simulink model "Calculate_average"  (R2021a)
settings: Solver=FixedStepDiscrete  StartTime=0.0  StopTime=10.0  RelTol=1e-3
settings Model: Creator=OmarMedhat  LastModifiedBy=OmarMedhat
settings OptimizationCC: DefaultParameterBehavior=Inlined  EnhancedBackFolding=on  PassReuseOutputArgsAs=Individual arguments  ZeroExternalMemoryAtStartup=off  ZeroInternalMemoryAtStartup=off  OptimizeBlockOrder=speed  DifferentSizesBufferReuse=on  OptimizationCustomize=off  EfficientTunableParamExpr=on
settings DebuggingCC: ParameterTunabilityLossMsg=error
settings SFSimCC: MATLABDynamicMemAlloc=off
settings RTWCC: SystemTargetFile=ert.tlc  GenCodeOnly=on  TemplateMakefile=ert_default_tmf  GenerateReport=on  IncludeHyperlinkInReport=on  LaunchReport=on  GenerateTraceInfo=on
settings CodeAppCC: ForceParamTrailComments=on  IgnoreCustomStorageClasses=off  OperatorAnnotations=on  SimulinkDataObjDesc=on  SFDataObjDesc=on  InsertBlockDesc=on
settings ERTTargetCC: TargetLangStandard=C99 (ISO)  GenerateSampleERTMain=on  InlinedParameterPlacement=NonHierarchical  ERTCustomFileTemplate=example_file_process.tlc

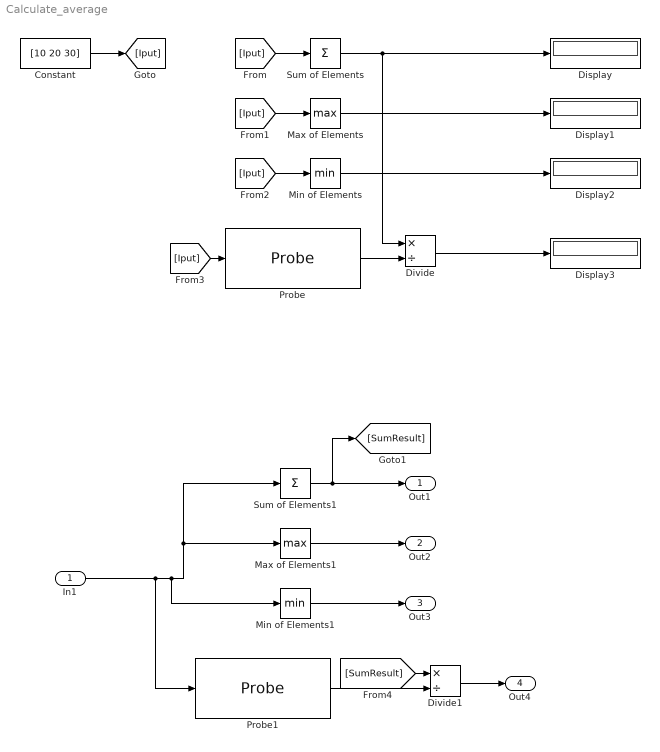
== system Calculate_average ==
  In1 : Inport  PortDimensions=10
  Constant : Constant  Value=[10 20 30]
  Display{,1..3} (4 alike) : Display
  Divide : Product  Inputs=*/
  Divide1 : Product  Inputs=*/
  Max of Elements : MinMax  Function=max
  Max of Elements1 : MinMax  Function=max
  Min of Elements : MinMax
  Min of Elements1 : MinMax
  Probe : Probe  ProbeSampleTime=off  ProbeComplexSignal=off
  Probe1 : Probe  ProbeSampleTime=off  ProbeComplexSignal=off
  Sum of Elements : Sum  Inputs=+
  Sum of Elements1 : Sum  Inputs=+
  Out1 : Outport
  Out2 : Outport  Port=2
  Out3 : Outport  Port=3
  Out4 : Outport  Port=4
  wires:
  Constant/1 -> [Iput]
  [Iput] -> Sum of Elements/1
  [Iput] -> Max of Elements/1
  [Iput] -> Min of Elements/1
  [Iput] -> Probe/1
  Probe/1 -> Divide/2
  Sum of Elements/1 -> Display/1, Divide/1
  Max of Elements/1 -> Display1/1
  Min of Elements/1 -> Display2/1
  Divide/1 -> Display3/1
  In1/1 -> Max of Elements1/1, Sum of Elements1/1, Min of Elements1/1, Probe1/1
  Probe1/1 -> Divide1/2
  Sum of Elements1/1 -> [SumResult], Out1/1
  [SumResult] -> Divide1/1
  Divide1/1 -> Out4/1
  Max of Elements1/1 -> Out2/1
  Min of Elements1/1 -> Out3/1
